simulink model "Bioreactor_for_olderversion_1_1"  (R2025a)
settings: Solver=VariableStepAuto  StartTime=0.0  StopTime=1500  RelTol=1e-3
libraries: simulink x1
settings Model: Creator=a  LastModifiedBy=sayed
settings OptimizationCC: BlockReduction=off  DefaultParameterBehavior=Inlined  BufferReuse=off

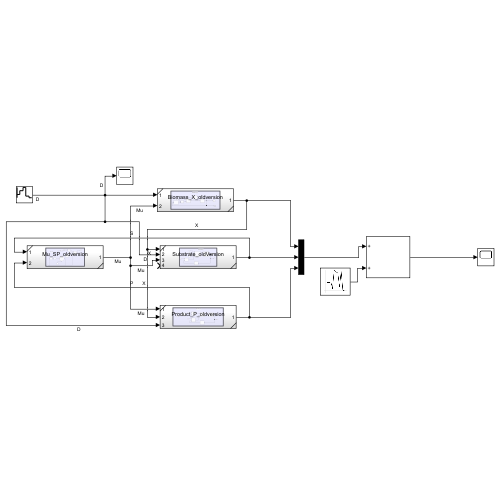
[thumbnail: Simulink's stored preview of the top-level diagram]
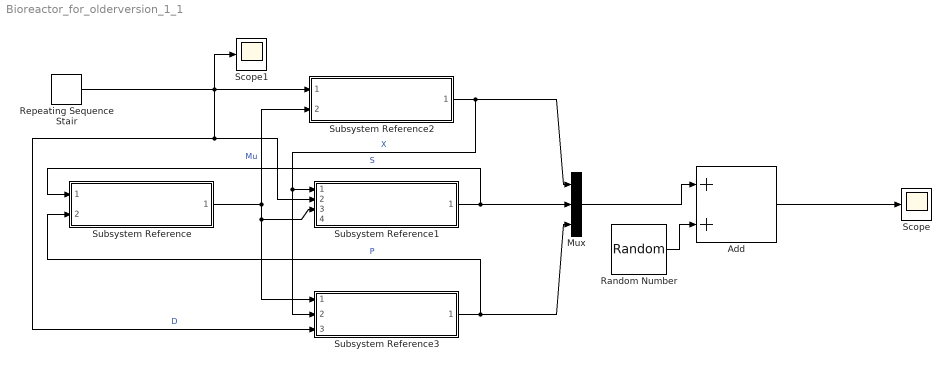
== system Bioreactor_for_olderversion_1_1 ==
  Add : Sum
  Mux : Mux  Inputs=3
  Random Number : RandomNumber  Variance=0.01  SampleTime=0.1
  Repeating Sequence Stair : simulink/Sources/Repeating Sequence Stair  OutValues=[0.202 0.2222 0.2424 0.1919 0.1818].'  tsamp=300  OutMin=[]  OutMax=[]  OutDataTypeStr=double  OutputDataTypeScalingMode=double  OutDataType=fixdt(0,8)  ConRadixGroup=Best Precision: Vector-wise  OutScaling=2^-12
  Scope : Scope
      settings: ActiveDisplayYMinimum=-2.8325448577427861  ActiveDisplayYMaximum=22.96147677624743
  Scope1 : Scope
      settings: ActiveDisplayYMinimum=-1  ActiveDisplayYMaximum=1
  Subsystem Reference : Subsystem  ReferencedSubsystem=Mu_SP_oldversion
  Subsystem Reference1 : Subsystem  ReferencedSubsystem=Substrate_oldVersion
  Subsystem Reference2 : Subsystem  ReferencedSubsystem=Biomass_X_oldversion
  Subsystem Reference3 : Subsystem  ReferencedSubsystem=Product_P_oldversion
  wires:
  Subsystem Reference/1 -> Subsystem Reference3/1, Subsystem Reference1/3, Subsystem Reference2/2  "Mu"
  Subsystem Reference2/1 -> Subsystem Reference3/2, Subsystem Reference1/1, Mux/1  "X"
  Subsystem Reference1/1 -> Mux/2, Subsystem Reference/1  "S"
  Subsystem Reference3/1 -> Subsystem Reference/2, Mux/3  "P"
  Repeating Sequence Stair/1 -> Scope1/1, Subsystem Reference3/3, Subsystem Reference1/2, Subsystem Reference2/1  "D"
  Mux/1 -> Add/1
  Random Number/1 -> Add/2
  Add/1 -> Scope/1
